simulink model "AMCLIB_BemfObsrvDQ_BAM_FLT"  (Simulink 8.3)
settings: Solver=ode45  StartTime=0.0  StopTime=10.0  RelTol=1e-3
undefined symbols (not defined in the file): fltCC1sc_D, fltCC1sc_Q, fltCC2sc_D, fltCC2sc_Q, fltEGain, fltIGain, fltLowerLimit_D, fltLowerLimit_Q, fltUGain, fltUpperLimit_D, fltUpperLimit_Q, fltWIGain
settings Model: Creator=B37097  LastModifiedBy=B37097
settings DataIOCC: SignalLoggingSaveFormat=Dataset
settings DebuggingCC: UnderspecifiedInitializationDetection=Simplified  StateNameClashWarn=none
settings GRTTargetCC: CombineOutputUpdateFcns=on  GRTInterface=off

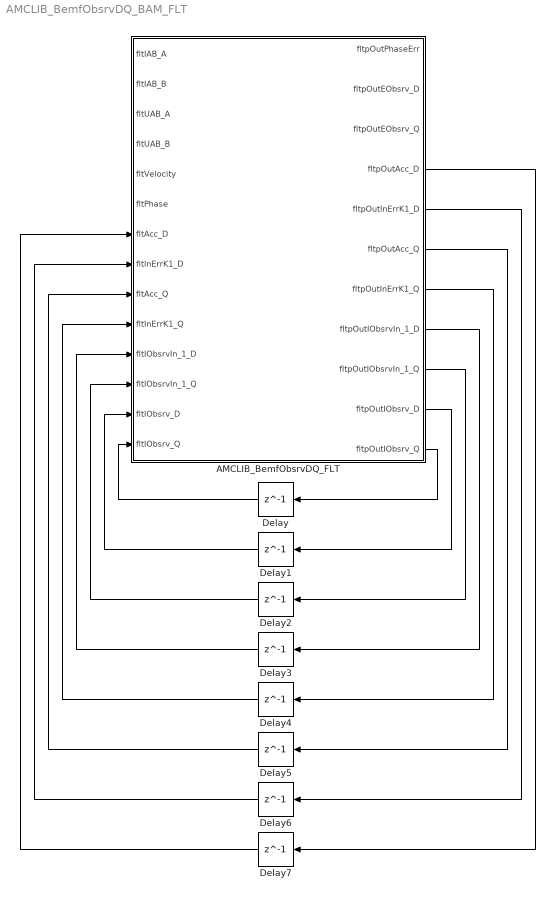
== system AMCLIB_BemfObsrvDQ_BAM_FLT ==
  AMCLIB_BemfObsrvDQ_FLT : Subsystem  mask(AMCLIB_BemfObsrvDQ_FLT){fltIGain=fltIGain, fltUGain=fltUGain, fltWIGain=fltWIGain, fltEGain=fltEGain, fltCC1sc_D=fltCC1sc_D, fltCC1sc_Q=fltCC1sc_Q, fltCC2sc_D=fltCC2sc_D, fltCC2sc_Q=fltCC2sc_Q, fltUpperLimit_D=fltUpperLimit_D, fltUpperLimit_Q=fltUpperLimit_Q, fltLowerLimit_D=fltLowerLimit_D, fltLowerLimit_Q=fltLowerLimit_Q}
      mask help: Bit accurate model of back-EMF observer DQ. All parameters as well as input and output values are in single precision floating data format.
      mask init:
      | pos = get_param(gcb, 'Position');width = pos(3) - pos(1); height = pos(4) - pos(2);tX=width/2;tY=height*0.9;
      mask Display: color('black');port_label('input',1,'fltIAB_A');port_label('input',2,'fltIAB_B');port_label('input',3,'fltUAB_A');port_label('input',4,'fltUAB_B');port_label('input',5,'fltVelocity');port_label('input',6,'fltPhase');port_label('input',7,'fltAcc_D');port_label('input',8,'fltInErrK1_D');port_label('input',9,'fltAcc_Q');port_label('input',10,'fltInErrK1_Q');port_label('input',11,'fltIObsrvIn_1_D');port_label('input',12,'fltIObsrvIn_1_Q');port_label('input',13,'fltIObsrv_D');port_label('input',14,'fltIObsrv_Q');port_label('output',1,'fltpOutPhaseErr');port_label('output',2,'fltpOutEObsrv_D');port_label('output',3,'fltpOutEObsrv_Q');port_label('output',4,'fltpOutAcc_D');port_label('output',5,'fltpOutInErrK1_D');port_label('output',6,'fltpOutAcc_Q');port_label('output',7,'fltpOutInErrK1_Q');port_label('output',8,'fltpOutIObsrvIn_1_D');port_label('output',9,'fltpOutIObsrvIn_1_Q');port_label('output',10,'fltpOutIObsrv_D');port_label('output',11,'fltpOutIObsrv_Q');color('black');disp('AMCLIB_BemfObsrvDQ_FLT');color('blue');text(tX,tY, 'BAM', 'horizontalAlignment', 'center');
  Delay{,1..7} (8 alike) : Delay  DelayLength=1  InitialCondition=0
  wires:
  AMCLIB_BemfObsrvDQ_FLT/11(fltpOutIObsrv_Q) -> Delay/1
  Delay/1 -> AMCLIB_BemfObsrvDQ_FLT/14(fltIObsrv_Q)
  AMCLIB_BemfObsrvDQ_FLT/10(fltpOutIObsrv_D) -> Delay1/1
  Delay1/1 -> AMCLIB_BemfObsrvDQ_FLT/13(fltIObsrv_D)
  AMCLIB_BemfObsrvDQ_FLT/9(fltpOutIObsrvIn_1_Q) -> Delay2/1
  Delay2/1 -> AMCLIB_BemfObsrvDQ_FLT/12(fltIObsrvIn_1_Q)
  AMCLIB_BemfObsrvDQ_FLT/8(fltpOutIObsrvIn_1_D) -> Delay3/1
  AMCLIB_BemfObsrvDQ_FLT/7(fltpOutInErrK1_Q) -> Delay4/1
  AMCLIB_BemfObsrvDQ_FLT/6(fltpOutAcc_Q) -> Delay5/1
  AMCLIB_BemfObsrvDQ_FLT/5(fltpOutInErrK1_D) -> Delay6/1
  AMCLIB_BemfObsrvDQ_FLT/4(fltpOutAcc_D) -> Delay7/1
  Delay3/1 -> AMCLIB_BemfObsrvDQ_FLT/11(fltIObsrvIn_1_D)
  Delay4/1 -> AMCLIB_BemfObsrvDQ_FLT/10(fltInErrK1_Q)
  Delay5/1 -> AMCLIB_BemfObsrvDQ_FLT/9(fltAcc_Q)
  Delay6/1 -> AMCLIB_BemfObsrvDQ_FLT/8(fltInErrK1_D)
  Delay7/1 -> AMCLIB_BemfObsrvDQ_FLT/7(fltAcc_D)

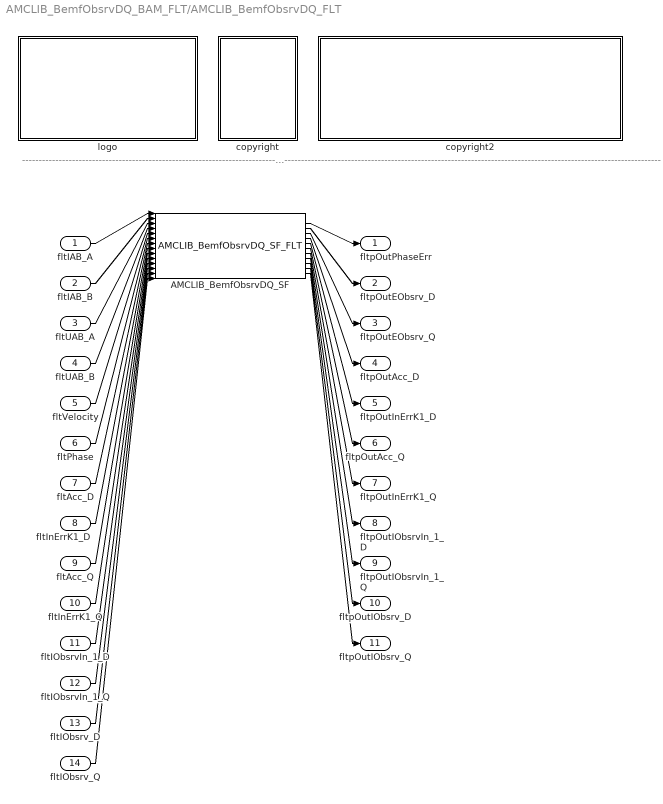
== system AMCLIB_BemfObsrvDQ_BAM_FLT/AMCLIB_BemfObsrvDQ_FLT ==
  note: ---------------------------------------------------------------------------------------------------------------------------------------------------------------------------------------------------
  fltIAB_A : Inport
  fltIAB_B : Inport  Port=2
  fltUAB_A : Inport  Port=3
  fltUAB_B : Inport  Port=4
  fltVelocity : Inport  Port=5
  fltPhase : Inport  Port=6
  fltAcc_D : Inport  Port=7
  fltInErrK1_D : Inport  Port=8
  fltAcc_Q : Inport  Port=9
  fltInErrK1_Q : Inport  Port=10
  fltIObsrvIn_1_D : Inport  Port=11
  fltIObsrvIn_1_Q : Inport  Port=12
  fltIObsrv_D : Inport  Port=13
  fltIObsrv_Q : Inport  Port=14
  AMCLIB_BemfObsrvDQ_SF : S-Function  FunctionName=AMCLIB_BemfObsrvDQ_SF_FLT  Parameters=fltIGain,fltUGain,fltWIGain,fltEGain,fltCC1sc_D,fltCC1sc_Q,fltCC2sc_D,fltCC2sc_Q,fltUpperLimit_D,fltUpperLimit_Q,fltLowerLimit_D,fltLowerLimit_Q  EnableBusSupport=off
  copyright : Subsystem
      mask Display: text(10,90,'FILE:');text(10,75,'DESRIPTION:');text(10,60,'COPYRIGHT:');text(10,45,'VERSION:');text(10,30,'DATE:')
  copyright2 : Subsystem
      mask Display: text(10,90,'AMCLIB_BemfObsrvDQ_BAM_FLT.mdl');text(10,75,'PMSM back-EMF observer DQ.');text(10,60,'NXP');text(10,45,'1.0');text(10,30,'26-Oct-2016');
  logo : Subsystem
      mask Display: image(imread('logo.jpg'))
  fltpOutPhaseErr : Outport
  fltpOutEObsrv_D : Outport  Port=2
  fltpOutEObsrv_Q : Outport  Port=3
  fltpOutAcc_D : Outport  Port=4
  fltpOutInErrK1_D : Outport  Port=5
  fltpOutAcc_Q : Outport  Port=6
  fltpOutInErrK1_Q : Outport  Port=7
  fltpOutIObsrvIn_1_D : Outport  Port=8
  fltpOutIObsrvIn_1_Q : Outport  Port=9
  fltpOutIObsrv_D : Outport  Port=10
  fltpOutIObsrv_Q : Outport  Port=11
  wires:
  fltIAB_A/1 -> AMCLIB_BemfObsrvDQ_SF/1
  fltIAB_B/1 -> AMCLIB_BemfObsrvDQ_SF/2
  fltUAB_A/1 -> AMCLIB_BemfObsrvDQ_SF/3
  fltUAB_B/1 -> AMCLIB_BemfObsrvDQ_SF/4
  fltVelocity/1 -> AMCLIB_BemfObsrvDQ_SF/5
  fltPhase/1 -> AMCLIB_BemfObsrvDQ_SF/6
  fltAcc_D/1 -> AMCLIB_BemfObsrvDQ_SF/7
  fltInErrK1_D/1 -> AMCLIB_BemfObsrvDQ_SF/8
  fltAcc_Q/1 -> AMCLIB_BemfObsrvDQ_SF/9
  fltInErrK1_Q/1 -> AMCLIB_BemfObsrvDQ_SF/10
  fltIObsrvIn_1_D/1 -> AMCLIB_BemfObsrvDQ_SF/11
  fltIObsrvIn_1_Q/1 -> AMCLIB_BemfObsrvDQ_SF/12
  fltIObsrv_D/1 -> AMCLIB_BemfObsrvDQ_SF/13
  fltIObsrv_Q/1 -> AMCLIB_BemfObsrvDQ_SF/14
  AMCLIB_BemfObsrvDQ_SF/1 -> fltpOutPhaseErr/1
  AMCLIB_BemfObsrvDQ_SF/2 -> fltpOutEObsrv_D/1
  AMCLIB_BemfObsrvDQ_SF/3 -> fltpOutEObsrv_Q/1
  AMCLIB_BemfObsrvDQ_SF/4 -> fltpOutAcc_D/1
  AMCLIB_BemfObsrvDQ_SF/5 -> fltpOutInErrK1_D/1
  AMCLIB_BemfObsrvDQ_SF/6 -> fltpOutAcc_Q/1
  AMCLIB_BemfObsrvDQ_SF/7 -> fltpOutInErrK1_Q/1
  AMCLIB_BemfObsrvDQ_SF/8 -> fltpOutIObsrvIn_1_D/1
  AMCLIB_BemfObsrvDQ_SF/9 -> fltpOutIObsrvIn_1_Q/1
  AMCLIB_BemfObsrvDQ_SF/10 -> fltpOutIObsrv_D/1
  AMCLIB_BemfObsrvDQ_SF/11 -> fltpOutIObsrv_Q/1

== system AMCLIB_BemfObsrvDQ_BAM_FLT/AMCLIB_BemfObsrvDQ_FLT/copyright ==

== system AMCLIB_BemfObsrvDQ_BAM_FLT/AMCLIB_BemfObsrvDQ_FLT/copyright2 ==

== system AMCLIB_BemfObsrvDQ_BAM_FLT/AMCLIB_BemfObsrvDQ_FLT/logo ==
